simulink library "UserContent_lib"  (Simulink 7.8)
settings: Solver=ode45  SolverMode=SingleTasking  StartTime=0.0  StopTime=10.0  RelTol=1e-3
undefined symbols (not defined in the file): bias, ln, Timestep, u_gain_light, u_gain_moderate, u_gain_severe, v_gain_light, v_gain_moderate, v_gain_severe, w_gain_light, w_gain_moderate, w_gain_severe, WindDir, WindSpd
libraries: simulink x8
(part 1 of 2)
settings Model: Creator=Austin Murch  LastModifiedBy=decox

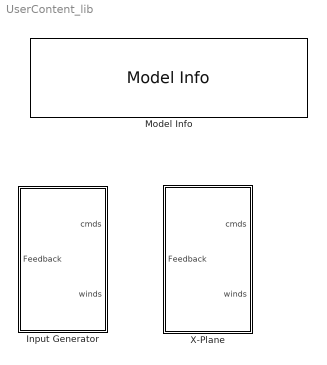
== system UserContent_lib ==
  Input Generator : Subsystem
  Model Info : simulink/Model-Wide Utilities/Model Info  InitialBlockCM=None  BlockCM=None  Frame=on  DisplayStringWithTags=|  HorizontalTextAlignment=Center  LeftAlignmentValue=0.5  SourceBlockDiagram=UserContent_lib  TagMaxNumber=20
      | - gtm_design Input Library -
      | 
      | Model Version: %<ModelVersion>
      | Last modifed by %<LastModifiedBy> on %<LastModificationDate>
  X-Plane : Subsystem

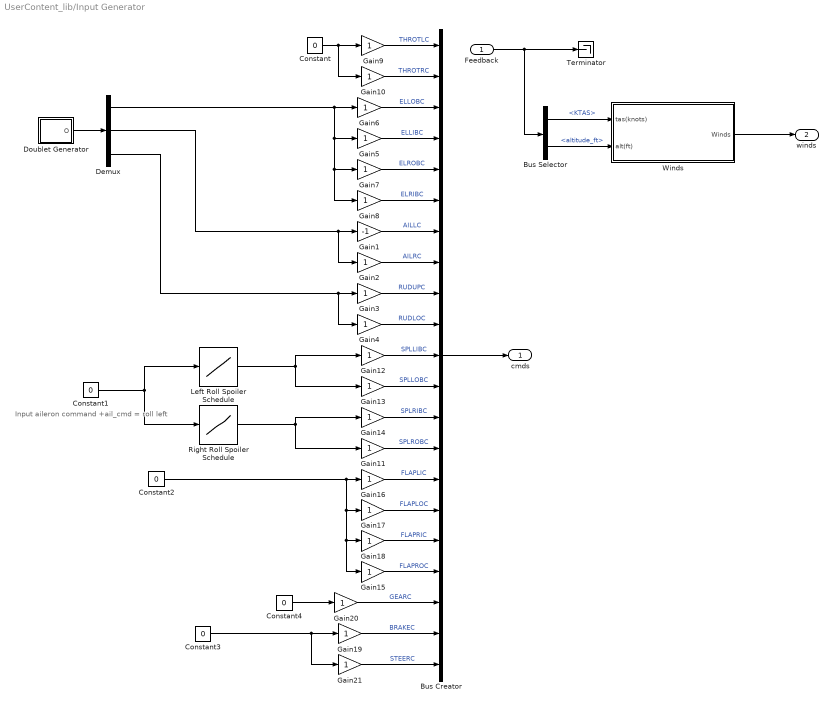
== system UserContent_lib/Input Generator ==
  note: Input aileron command
      | +ail_cmd = roll left
  Feedback : Inport
  Bus Creator : BusCreator  Inputs=21
  Bus Selector : BusSelector  OutputSignals=AirData.KTAS,AirData.altitude_ft
  Constant{,1..4} (5 alike) : Constant  Value=0
  Demux : Demux  Outputs=3
  Doublet Generator : Subsystem  mask(DoubletGenerator){timeon=[2 12 7], pulsewidth=[0.5 0.5 0.5], amplitude=[0 0 0]}
      mask prompts: timeon "Time Start"; pulsewidth "Pulse Duration"
      mask help:
      | Doublet Generator.
      | Ouputs doublet of specificed amplitude and duration.
      |
      | If start/duration/amplitude parameters are vectors, then output is multichannel.
      mask Display: plot([.1 .3 .3001 .4 .4001 .5  .5001 .7],[0 0 1 1 -1 -1 0 0])
  Gain1 : Gain  Gain=-1  SaturateOnIntegerOverflow=on  OutDataTypeStr=Inherit: Same as input  ParamDataTypeStr=Inherit: Same as input
  Gain{2..21} (20 alike) : Gain  SaturateOnIntegerOverflow=on  OutDataTypeStr=Inherit: Same as input  ParamDataTypeStr=Inherit: Same as input
  Left Roll Spoiler Schedule : Lookup  InputValues="[-20\t-11.76\t-2.36\t0\t2.36\t11.76\t20\t]"  Table=[0 0 0 0 0 9 45]  LookUpMeth=Interpolation-Use End Values
  Right Roll Spoiler Schedule : Lookup  InputValues="[-20\t-11.76\t-2.36\t0\t2.36\t11.76\t20\t]"  Table=[45 9 0 0 0 0 0]  LookUpMeth=Interpolation-Use End Values
  Terminator : Terminator
  Winds : Subsystem  mask(WindSource){WindSpeed_knots=WindSpd, WindDirection_deg=WindDir, level=None}
      mask prompts: WindSpeed_knots "Wind Speed (knots)"; WindDirection_deg "Wind Direction (deg)"; level "Turbulence Level"
      mask help:
      | Sets steady winds with wind speed and direction and
      | applies gust winds with selectable level of turbulence.
      mask StyleString: edit,edit,popup(None|Light|Moderate|Severe)
  cmds : Outport
  winds : Outport  Port=2
  wires:
  Winds/1(Winds) -> winds/1
  Constant1/1 -> Right Roll Spoiler Schedule/1, Left Roll Spoiler Schedule/1
  Right Roll Spoiler Schedule/1 -> Gain11/1, Gain14/1
  Left Roll Spoiler Schedule/1 -> Gain13/1, Gain12/1
  Gain12/1 -> Bus Creator/11  "SPLLIBC"
  Gain13/1 -> Bus Creator/12  "SPLLOBC"
  Gain14/1 -> Bus Creator/13  "SPLRIBC"
  Gain11/1 -> Bus Creator/14  "SPLROBC"
  Gain16/1 -> Bus Creator/15  "FLAPLIC"
  Gain17/1 -> Bus Creator/16  "FLAPLOC"
  Gain18/1 -> Bus Creator/17  "FLAPRIC"
  Gain15/1 -> Bus Creator/18  "FLAPROC"
  Gain9/1 -> Bus Creator/1  "THROTLC"
  Gain10/1 -> Bus Creator/2  "THROTRC"
  Gain5/1 -> Bus Creator/4  "ELLIBC"
  Gain6/1 -> Bus Creator/3  "ELLOBC"
  Gain7/1 -> Bus Creator/5  "ELROBC"
  Gain8/1 -> Bus Creator/6  "ELRIBC"
  Gain1/1 -> Bus Creator/7  "AILLC"
  Gain2/1 -> Bus Creator/8  "AILRC"
  Gain3/1 -> Bus Creator/9  "RUDUPC"
  Gain4/1 -> Bus Creator/10  "RUDLOC"
  Constant/1 -> Gain10/1, Gain9/1
  Constant2/1 -> Gain16/1, Gain17/1, Gain18/1, Gain15/1
  Doublet Generator/1(O) -> Demux/1
  Demux/2 -> Gain1/1, Gain2/1
  Demux/3 -> Gain3/1, Gain4/1
  Gain19/1 -> Bus Creator/20  "BRAKEC"
  Constant4/1 -> Gain20/1
  Constant3/1 -> Gain19/1, Gain21/1
  Demux/1 -> Gain6/1, Gain5/1, Gain7/1, Gain8/1
  Bus Creator/1 -> cmds/1
  Gain20/1 -> Bus Creator/19  "GEARC"
  Gain21/1 -> Bus Creator/21  "STEERC"
  Feedback/1 -> Terminator/1, Bus Selector/1
  Bus Selector/1 -> Winds/1(tas(knots))  "<KTAS>"
  Bus Selector/2 -> Winds/2(alt(ft))  "<altitude_ft>"

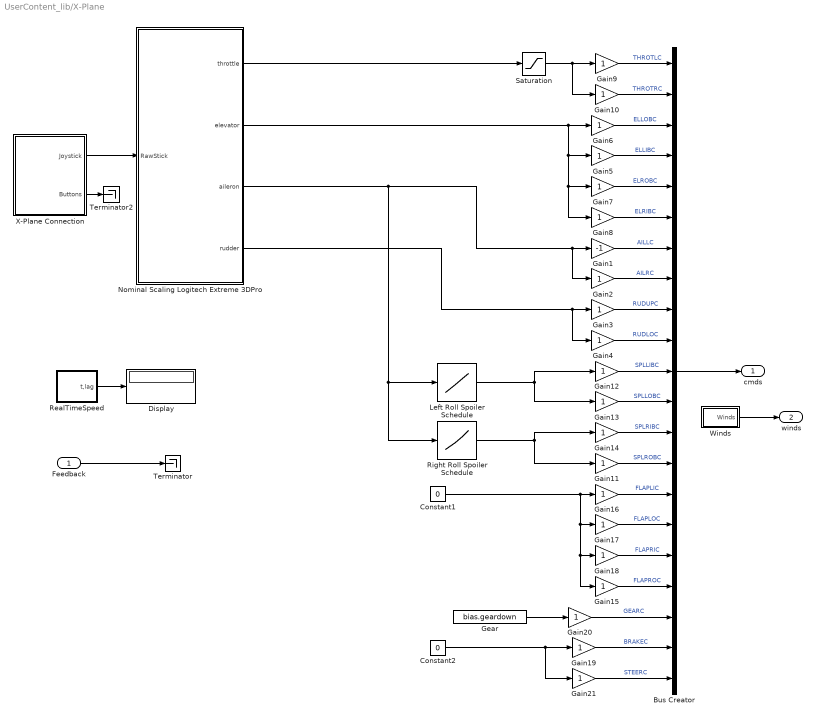
== system UserContent_lib/X-Plane ==
  Feedback : Inport
  Bus Creator : BusCreator  Inputs=21
  Constant1 : Constant  Value=0
  Constant2 : Constant  Value=0
  Display : Display
  Gain1 : Gain  Gain=-1  SaturateOnIntegerOverflow=on  OutDataTypeStr=Inherit: Same as input  ParamDataTypeStr=Inherit: Same as input
  Gain{2..21} (20 alike) : Gain  SaturateOnIntegerOverflow=on  OutDataTypeStr=Inherit: Same as input  ParamDataTypeStr=Inherit: Same as input
  Gear : Constant  Value=bias.geardown
  Left Roll Spoiler Schedule : Lookup  InputValues="[-20\t-11.76\t-2.36\t0\t2.36\t11.76\t20\t]"  Table=[0 0 0 0 0 9 45]  LookUpMeth=Interpolation-Use End Values
  Nominal Scaling Logitech Extreme 3DPro : Subsystem
  RealTimeSpeed : Subsystem
  Right Roll Spoiler Schedule : Lookup  InputValues="[-20\t-11.76\t-2.36\t0\t2.36\t11.76\t20\t]"  Table=[45 9 0 0 0 0 0]  LookUpMeth=Interpolation-Use End Values
  Saturation : Saturate  UpperLimit=100  LowerLimit=0
  Terminator : Terminator
  Terminator2 : Terminator
  Winds : Subsystem
  X-Plane Connection : Subsystem
  cmds : Outport
  winds : Outport  Port=2
  wires:
  Nominal Scaling Logitech Extreme 3DPro/1(throttle) -> Saturation/1
  Nominal Scaling Logitech Extreme 3DPro/2(elevator) -> Gain6/1, Gain5/1, Gain7/1, Gain8/1
  Nominal Scaling Logitech Extreme 3DPro/3(aileron) -> Right Roll Spoiler Schedule/1, Left Roll Spoiler Schedule/1, Gain1/1, Gain2/1
  Nominal Scaling Logitech Extreme 3DPro/4(rudder) -> Gain3/1, Gain4/1
  X-Plane Connection/2(Buttons) -> Terminator2/1
  Saturation/1 -> Gain10/1, Gain9/1
  RealTimeSpeed/1(t,lag) -> Display/1
  X-Plane Connection/1(Joystick) -> Nominal Scaling Logitech Extreme 3DPro/1(RawStick)
  Gain12/1 -> Bus Creator/11  "SPLLIBC"
  Gain13/1 -> Bus Creator/12  "SPLLOBC"
  Gain14/1 -> Bus Creator/13  "SPLRIBC"
  Gain11/1 -> Bus Creator/14  "SPLROBC"
  Gain16/1 -> Bus Creator/15  "FLAPLIC"
  Gain17/1 -> Bus Creator/16  "FLAPLOC"
  Gain18/1 -> Bus Creator/17  "FLAPRIC"
  Gain15/1 -> Bus Creator/18  "FLAPROC"
  Gain9/1 -> Bus Creator/1  "THROTLC"
  Gain10/1 -> Bus Creator/2  "THROTRC"
  Gain5/1 -> Bus Creator/4  "ELLIBC"
  Gain6/1 -> Bus Creator/3  "ELLOBC"
  Gain7/1 -> Bus Creator/5  "ELROBC"
  Gain8/1 -> Bus Creator/6  "ELRIBC"
  Gain1/1 -> Bus Creator/7  "AILLC"
  Gain2/1 -> Bus Creator/8  "AILRC"
  Gain3/1 -> Bus Creator/9  "RUDUPC"
  Gain4/1 -> Bus Creator/10  "RUDLOC"
  Constant1/1 -> Gain16/1, Gain17/1, Gain18/1, Gain15/1
  Gain19/1 -> Bus Creator/20  "BRAKEC"
  Gear/1 -> Gain20/1
  Constant2/1 -> Gain19/1, Gain21/1
  Bus Creator/1 -> cmds/1
  Gain20/1 -> Bus Creator/19  "GEARC"
  Gain21/1 -> Bus Creator/21  "STEERC"
  Left Roll Spoiler Schedule/1 -> Gain12/1, Gain13/1
  Right Roll Spoiler Schedule/1 -> Gain14/1, Gain11/1
  Feedback/1 -> Terminator/1
  Winds/1(Winds) -> winds/1

== system UserContent_lib/Input Generator/Doublet Generator ==
  Add : Sum  Inputs=+++
  DownStep : Step  Time=timeon+pulsewidth  After=-2  SampleTime=0
  Gain : Gain  Gain=amplitude
  UnStep : Step  Time=timeon+2*pulsewidth  SampleTime=0
  UpStep : Step  Time=timeon  SampleTime=0
  O : Outport
  wires:
  UpStep/1 -> Add/1
  DownStep/1 -> Add/2
  UnStep/1 -> Add/3
  Add/1 -> Gain/1
  Gain/1 -> O/1

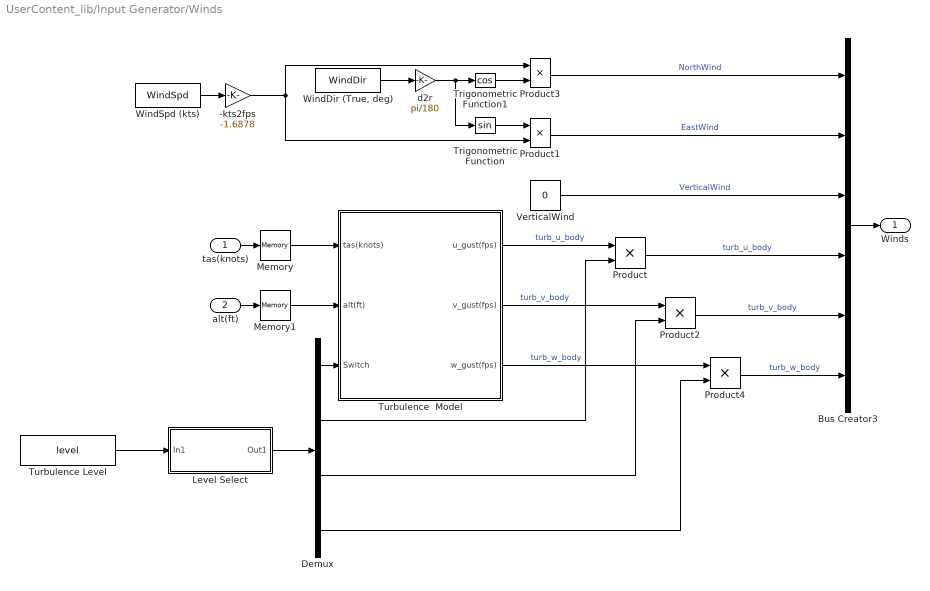
== system UserContent_lib/Input Generator/Winds ==
  tas(knots) : Inport
  alt(ft) : Inport  Port=2
  -kts2fps : Gain  Gain=-1.6878  SaturateOnIntegerOverflow=on  OutDataTypeStr=Inherit: Same as input  ParamDataTypeStr=Inherit: Same as input
  Bus Creator3 : BusCreator  Inputs=6
  Demux : Demux
  Level Select : Subsystem
  Memory : Memory  X0=70
  Memory1 : Memory  X0=1000
  Product : Product  RndMeth=Zero
  Product1 : Product  Inputs=**  SaturateOnIntegerOverflow=on  InputSameDT=on  OutDataTypeStr=Inherit: Same as first input
  Product2 : Product  RndMeth=Zero
  Product3 : Product  Inputs=**  SaturateOnIntegerOverflow=on  InputSameDT=on  OutDataTypeStr=Inherit: Same as first input
  Product4 : Product  RndMeth=Zero
  Trigonometric Function : Trigonometry
  Trigonometric Function1 : Trigonometry  Operator=cos
  Turbulence  Model : Subsystem
  Turbulence Level : Constant  Value=level
  VerticalWind : Constant  Value=0
  "WindDir (True, deg)" : Constant  Value=WindDir
  WindSpd (kts) : Constant  Value=WindSpd
  d2r : Gain  Gain=pi/180  SaturateOnIntegerOverflow=on  OutDataTypeStr=Inherit: Same as input  ParamDataTypeStr=Inherit: Same as input
  Winds : Outport
  wires:
  Demux/4 -> Product4/2
  Demux/3 -> Product2/2
  Demux/2 -> Product/2
  Demux/1 -> Turbulence  Model/3(Switch)
  Product3/1 -> Bus Creator3/1  "NorthWind"
  Product1/1 -> Bus Creator3/2  "EastWind"
  VerticalWind/1 -> Bus Creator3/3  "VerticalWind"
  Bus Creator3/1 -> Winds/1
  Trigonometric Function/1 -> Product1/1
  Trigonometric Function1/1 -> Product3/2
  d2r/1 -> Trigonometric Function1/1, Trigonometric Function/1
  "WindDir (True, deg)"/1 -> d2r/1
  WindSpd (kts)/1 -> -kts2fps/1
  -kts2fps/1 -> Product1/2, Product3/1
  Turbulence  Model/1(u_gust(fps)) -> Product/1  "turb_u_body"
  Turbulence  Model/2(v_gust(fps)) -> Product2/1  "turb_v_body"
  Turbulence  Model/3(w_gust(fps)) -> Product4/1  "turb_w_body"
  Product/1 -> Bus Creator3/4  "turb_u_body"
  Product2/1 -> Bus Creator3/5  "turb_v_body"
  Product4/1 -> Bus Creator3/6  "turb_w_body"
  tas(knots)/1 -> Memory/1
  alt(ft)/1 -> Memory1/1
  Memory/1 -> Turbulence  Model/1(tas(knots))
  Memory1/1 -> Turbulence  Model/2(alt(ft))
  Turbulence Level/1 -> Level Select/1(In1)
  Level Select/1(Out1) -> Demux/1

== system UserContent_lib/X-Plane/Nominal Scaling Logitech Extreme 3DPro ==
  RawStick : Inport
  Bias : Bias  Bias=[-1 -.5 -.5 -.5]
  Clock : Clock
  Constant : Constant  Value=zeros(4,1)
  Demux : Demux  Outputs=[4 -1]
  Demux1 : Demux
  Gain : Gain  Gain=[-100 -15 -15 -15]
  InitiallSupress Stick ToAllowTrim : Switch  Threshold=0.25
  Memory : Memory  X0=zeros(16,1)
  Selector : Selector  InputPortWidth=4  IndexOptions=Index vector (dialog)  Indices=[4 2 1 3]  OutputSizes=1
  Terminator3 : Terminator
  throttle : Outport
  elevator : Outport  Port=2
  aileron : Outport  Port=3
  rudder : Outport  Port=4
  wires:
  Demux1/4 -> rudder/1
  Demux1/3 -> aileron/1
  Demux1/2 -> elevator/1
  Demux1/1 -> throttle/1
  InitiallSupress Stick ToAllowTrim/1 -> Demux1/1
  Clock/1 -> InitiallSupress Stick ToAllowTrim/2
  Constant/1 -> InitiallSupress Stick ToAllowTrim/3
  Gain/1 -> InitiallSupress Stick ToAllowTrim/1
  Selector/1 -> Bias/1
  Bias/1 -> Gain/1
  RawStick/1 -> Memory/1
  Memory/1 -> Demux/1
  Demux/2 -> Terminator3/1
  Demux/1 -> Selector/1

== system UserContent_lib/X-Plane/RealTimeSpeed ==
  Clock : Clock
  Demux : Demux  Outputs=2
  Mux : Mux  Inputs=2
  S-Function : S-Function  FunctionName=RT_mex  EnableBusSupport=off
  Subtract : Sum  Inputs=+-
  t,lag : Outport
  wires:
  Mux/1 -> t,lag/1
  Subtract/1 -> Mux/2
  Demux/2 -> Subtract/2
  Demux/1 -> Mux/1, Subtract/1
  S-Function/1 -> Demux/1
  Clock/1 -> S-Function/1

== system UserContent_lib/X-Plane/Winds ==
  -kts2fps : Gain  Gain=-1.6878  SaturateOnIntegerOverflow=on  OutDataTypeStr=Inherit: Same as input  ParamDataTypeStr=Inherit: Same as input
  Bus Creator3 : BusCreator  Inputs=6
  Product1 : Product  Inputs=**  SaturateOnIntegerOverflow=on  InputSameDT=on  OutDataTypeStr=Inherit: Same as first input
  Product3 : Product  Inputs=**  SaturateOnIntegerOverflow=on  InputSameDT=on  OutDataTypeStr=Inherit: Same as first input
  Trigonometric Function : Trigonometry
  Trigonometric Function1 : Trigonometry  Operator=cos
  VerticalWind : Constant  Value=0
  "WindDir (True, deg)" : Constant  Value=WindDir
  WindSpd (kts) : Constant  Value=WindSpd
  d2r : Gain  Gain=pi/180  SaturateOnIntegerOverflow=on  OutDataTypeStr=Inherit: Same as input  ParamDataTypeStr=Inherit: Same as input
  turb_v_body : Constant  Value=0
  turb_v_body1 : Constant  Value=0
  turb_w_body : Constant  Value=0
  Winds : Outport
  wires:
  Product3/1 -> Bus Creator3/1  "NorthWind"
  Product1/1 -> Bus Creator3/2  "EastWind"
  VerticalWind/1 -> Bus Creator3/3  "VerticalWind"
  Bus Creator3/1 -> Winds/1
  Trigonometric Function/1 -> Product1/1
  Trigonometric Function1/1 -> Product3/2
  d2r/1 -> Trigonometric Function/1, Trigonometric Function1/1
  "WindDir (True, deg)"/1 -> d2r/1
  WindSpd (kts)/1 -> -kts2fps/1
  -kts2fps/1 -> Product3/1, Product1/2
  turb_v_body1/1 -> Bus Creator3/4  "turb_u_body"
  turb_v_body/1 -> Bus Creator3/5  "turb_v_body"
  turb_w_body/1 -> Bus Creator3/6  "turb_w_body"

== system UserContent_lib/X-Plane/X-Plane Connection ==
  Bus Selector1 : BusSelector  OutputSignals=AILR,ELRIB,RUDU,FLAPRIB,GEAR,BRAKE  OutputAsBus=on
  Bus Selector5 : BusSelector  OutputSignals=latitude,longitude,altitude,phi,theta,psi  OutputAsBus=on
  Bus Selector6 : BusSelector  OutputSignals=alpha,beta,tas  OutputAsBus=on
  Bus to Vector : BusToVector
  Bus to Vector1 : BusToVector
  Bus to Vector2 : BusToVector
  Xlink_fcn : Subsystem  mask(Xlink){HUDCell={'alpha','beta','Velocity'}}
      mask prompts: HUDCell "Lables for HUD, (cell array)"
      mask help:
      | Input Positions and Surfaces for X-Plane Visualization.
      |   Positions - [ Latitude, Longitude, Altitude, Roll, Pitch, Yaw] % degrees and ft.
      |   Surfaces  - [ Aileron, Elevator, Rudder, Flaps, Spoiler, GearDown] % deg and 0/1
      |
      | Output is Joysick axes and Button pushes.
      |   Joystick - First 16 axes
      |   Buttons  - 16 buttons as assigned to Xlink in X-Plane
      mask init:
      | if isempty(HUDCell) HUDCell=cell(6,1); end
      | HUDTextArray = uint8(zeros(90,1));
      | 
      | % loop through names, assign to string arrays
      | for i=1:min(length(HUDCell),6);
      |   if length(HUDCell{i})>14 HUDCell{i}=HUDCell{i}(1:14); end
      |   if length(HUDCell{i}>0),
      |     HUDTextArray((i-1)*15+1:(i-1)*15+length(HUDCell{i})) = uint8(HUDCell{i});
      |   end
      | end
  rad2deg : Gain  Gain=[180/pi 180/pi 1 180/pi 180/pi 180/pi]
  Joystick : Outport
  Buttons : Outport  Port=2
  wires:
  Bus Selector1/1 -> Bus to Vector1/1
  Bus to Vector1/1 -> Xlink_fcn/2(Surfaces)
  [SurfacePos] -> Bus Selector1/1
  rad2deg/1 -> Xlink_fcn/1(Positions)
  [EOM_State] -> Bus Selector5/1
  [AuxVars] -> Bus Selector6/1
  Bus Selector5/1 -> Bus to Vector2/1
  Xlink_fcn/2(Buttons) -> Buttons/1
  Xlink_fcn/1(Joystick) -> Joystick/1
  Bus Selector6/1 -> Bus to Vector/1
  Bus to Vector/1 -> Xlink_fcn/3(Overlay)
  Bus to Vector2/1 -> rad2deg/1

== system UserContent_lib/Input Generator/Winds/Level Select ==
  In1 : Inport
  Light : Constant  Value=[1 u_gain_light v_gain_light w_gain_light]
  Moderate : Constant  Value=[1 u_gain_moderate v_gain_moderate w_gain_moderate]
  Multiport Switch : MultiPortSwitch  Inputs=4  zeroidx=off
  Severe : Constant  Value=[1 u_gain_severe v_gain_severe w_gain_severe]
  Turbulence Off : Constant  Value=[0 0 0 0]
  Out1 : Outport
  wires:
  In1/1 -> Multiport Switch/1
  Turbulence Off/1 -> Multiport Switch/2
  Light/1 -> Multiport Switch/3
  Moderate/1 -> Multiport Switch/4
  Severe/1 -> Multiport Switch/5
  Multiport Switch/1 -> Out1/1

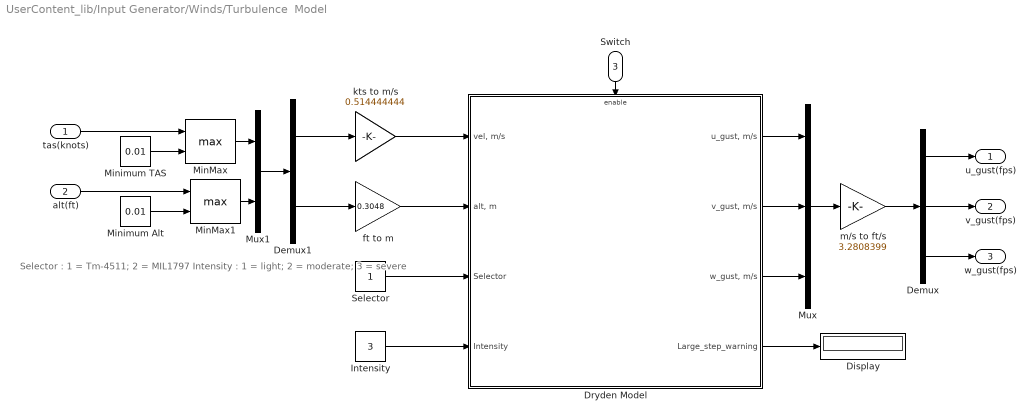
== system UserContent_lib/Input Generator/Winds/Turbulence  Model ==
  note: Selector :  1 = Tm-4511;  2 = MIL1797
      |             Intensity :  1 = light;  2 = moderate;  3 = severe
  tas(knots) : Inport
  alt(ft) : Inport  Port=2
  Switch : Inport  Port=3
  Demux : Demux  Outputs=3
  Demux1 : Demux  Outputs=2
  Display : Display
  Dryden Model : Subsystem  mask{longseed=3366+521, latseed=23+521, vertseed=1369+521, dt=Timestep, Step_warning_pct=.11}
      mask prompts: longseed "Longitudinal Random Number Seed"; latseed "Lateral Random Number Seed"; vertseed "Vertical Random Number Seed"; dt "Turbulence model time step, sec"; Step_warning_pct "Threshhold for stepsize warning (%)"
  Intensity : Constant  Value=3
  MinMax : MinMax  Function=max  Inputs=2
  MinMax1 : MinMax  Function=max  Inputs=2
  Minimum Alt : Constant  Value=0.01
  Minimum TAS : Constant  Value=0.01
  Mux : Mux  Inputs=3
  Mux1 : Mux  Inputs=2
  Selector : Constant
  ft to m : Gain  Gain=0.3048
  kts to m/s : Gain  Gain=0.514444444
  m/s to ft/s : Gain  Gain=3.2808399
  u_gust(fps) : Outport
  v_gust(fps) : Outport  Port=2
  w_gust(fps) : Outport  Port=3
  wires:
  Switch/1 -> Dryden Model/Enable
  Dryden Model/1("u_gust, m/s") -> Mux/1
  Dryden Model/2("v_gust, m/s") -> Mux/2
  Dryden Model/3("w_gust, m/s") -> Mux/3
  Demux/3 -> w_gust(fps)/1
  Demux/2 -> v_gust(fps)/1
  Demux/1 -> u_gust(fps)/1
  Dryden Model/4(Large_step_warning) -> Display/1
  Mux/1 -> m/s to ft/s/1
  m/s to ft/s/1 -> Demux/1
  MinMax1/1 -> Mux1/2
  MinMax/1 -> Mux1/1
  alt(ft)/1 -> MinMax1/1
  Minimum Alt/1 -> MinMax1/2
  Minimum TAS/1 -> MinMax/2
  tas(knots)/1 -> MinMax/1
  Mux1/1 -> Demux1/1
  Demux1/2 -> ft to m/1
  Demux1/1 -> kts to m/s/1
  Intensity/1 -> Dryden Model/4(Intensity)
  Selector/1 -> Dryden Model/3(Selector)
  ft to m/1 -> Dryden Model/2("alt, m")
  kts to m/s/1 -> Dryden Model/1("vel, m/s")

== system UserContent_lib/X-Plane/X-Plane Connection/Xlink_fcn ==
  note: Force Input to
      | dimension 6
  Positions : Inport
  Surfaces : Inport  Port=2
  Overlay : Inport  Port=3
  Demux : Demux  Outputs=[6 -1]
  Labels : Constant  Value=HUDTextArray  OutDataTypeStr=uint8
  Mux : Mux  Inputs=2
  S-Function : S-Function  FunctionName=SimulinkToXPlane  EnableBusSupport=off
  Saturation : Saturate  UpperLimit=[180*ones(5,1); 1]  LowerLimit=[-180*ones(5,1); 0]
  Signal Specification3 : SignalSpecification  Dimensions=6
  Terminator : Terminator
  zeros : Constant  Value=zeros(6,1)  OutDataTypeStr=double
  Joystick : Outport
  Buttons : Outport  Port=2
  wires:
  Demux/2 -> Terminator/1
  Demux/1 -> Signal Specification3/1
  Mux/1 -> Demux/1
  zeros/1 -> Mux/2
  Overlay/1 -> Mux/1
  Labels/1 -> S-Function/3
  Saturation/1 -> S-Function/2
  S-Function/2 -> Buttons/1
  Surfaces/1 -> Saturation/1
  S-Function/1 -> Joystick/1
  Positions/1 -> S-Function/1
  Signal Specification3/1 -> S-Function/4

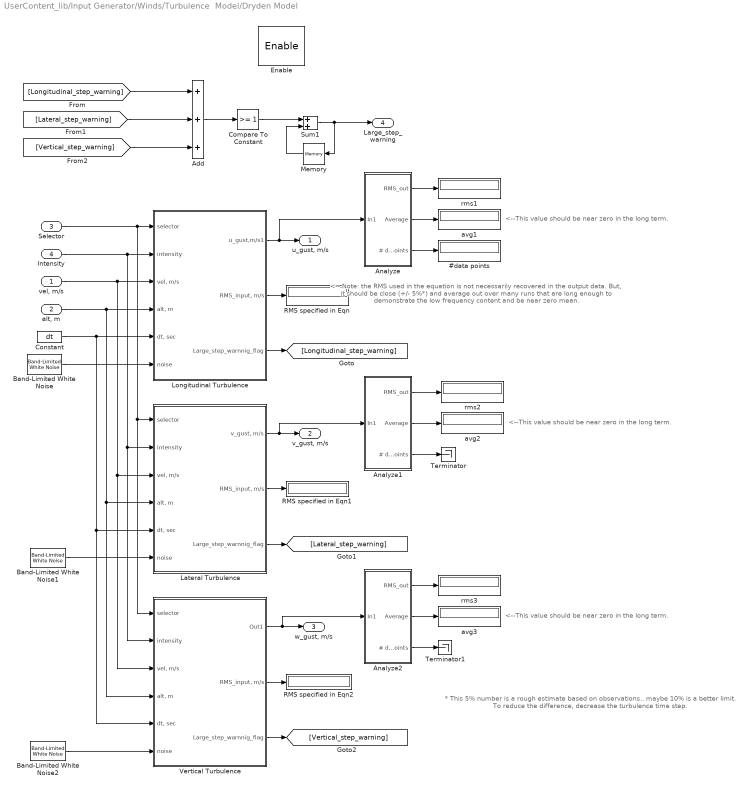
== system UserContent_lib/Input Generator/Winds/Turbulence  Model/Dryden Model ==
  note: * This 5% number is a rough estimate based on observations.. maybe 10% is a better limit.
      | To reduce the difference, decrease the turbulence time step.
  note: <--This value should be near zero in the long term.
  note: <--This value should be near zero in the long term.
  note: <--This value should be near zero in the long term.
  note: <-- Note: the RMS used in the equation is not necessarily recovered
      | in the output data.  But, it should be close (+/- 5%*) and  average out over
      | many runs that are long enough to demonstrate the low frequency
      | content and be near zero mean.
  "vel, m/s" : Inport
  "alt, m" : Inport  Port=2
  Selector : Inport  Port=3
  Intensity : Inport  Port=4
  Enable : EnablePort  StatesWhenEnabling=reset
  #data points : Display
  Add : Sum  Inputs=3
  Analyze : Subsystem
  Analyze1 : Subsystem
  Analyze2 : Subsystem
  Band-Limited White Noise : simulink/Sources/Band-Limited White Noise  Cov=dt  Ts=dt  seed=longseed
  Band-Limited White Noise1 : simulink/Sources/Band-Limited White Noise  Cov=dt  Ts=dt  seed=latseed
  Band-Limited White Noise2 : simulink/Sources/Band-Limited White Noise  Cov=dt  Ts=dt  seed=vertseed
  Compare To Constant : simulink/Logic and Bit Operations/Compare To Constant  relop=>=  const=1  OutDataTypeStr=uint8  ZeroCross=off
  Constant : Constant  Value=dt
  Lateral Turbulence : Subsystem
  Longitudinal Turbulence : Subsystem
  Memory : Memory
  RMS specified in Eqn : Display
  RMS specified in Eqn1 : Display
  RMS specified in Eqn2 : Display
  Sum1 : Sum  Inputs=2  SaturateOnIntegerOverflow=on
  Terminator : Terminator
  Terminator1 : Terminator
  Vertical Turbulence : Subsystem
  avg1 : Display
  avg2 : Display
  avg3 : Display
  rms1 : Display
  rms2 : Display
  rms3 : Display
  "u_gust, m/s" : Outport  OutputWhenDisabled=reset  InitialOutput=0
  "v_gust, m/s" : Outport  Port=2  OutputWhenDisabled=reset  InitialOutput=0
  "w_gust, m/s" : Outport  Port=3  OutputWhenDisabled=reset  InitialOutput=0
  Large_step_warning : Outport  Port=4  OutputWhenDisabled=reset  InitialOutput=0
  wires:
  Sum1/1 -> Memory/1, Large_step_warning/1
  Memory/1 -> Sum1/2
  Compare To Constant/1 -> Sum1/1
  Vertical Turbulence/3(Large_step_warnnig_flag) -> [Vertical_step_warning]
  Lateral Turbulence/3(Large_step_warnnig_flag) -> [Lateral_step_warning]
  Longitudinal Turbulence/3(Large_step_warnnig_flag) -> [Longitudinal_step_warning]
  [Lateral_step_warning] -> Add/2
  [Vertical_step_warning] -> Add/3
  [Longitudinal_step_warning] -> Add/1
  Add/1 -> Compare To Constant/1
  Band-Limited White Noise/1 -> Longitudinal Turbulence/6(noise)
  Analyze2/3(# data points) -> Terminator1/1
  Analyze1/3(# data points) -> Terminator/1
  Analyze/3(# data points) -> #data points/1
  Vertical Turbulence/2("RMS_input, m/s") -> RMS specified in Eqn2/1
  Lateral Turbulence/2("RMS_input, m/s") -> RMS specified in Eqn1/1
  Longitudinal Turbulence/2("RMS_input, m/s") -> RMS specified in Eqn/1
  Analyze2/2(Average) -> avg3/1
  Analyze2/1(RMS_out) -> rms3/1
  Vertical Turbulence/1(Out1) -> Analyze2/1(In1), "w_gust, m/s"/1
  Analyze1/2(Average) -> avg2/1
  Analyze1/1(RMS_out) -> rms2/1
  Lateral Turbulence/1("v_gust, m/s") -> Analyze1/1(In1), "v_gust, m/s"/1
  Analyze/2(Average) -> avg1/1
  Longitudinal Turbulence/1(u_gust,m/s1) -> Analyze/1(In1), "u_gust, m/s"/1
  Analyze/1(RMS_out) -> rms1/1
  Intensity/1 -> Lateral Turbulence/2(intensity), Vertical Turbulence/2(intensity), Longitudinal Turbulence/2(intensity)
  Band-Limited White Noise2/1 -> Vertical Turbulence/6(noise)
  Selector/1 -> Lateral Turbulence/1(selector), Vertical Turbulence/1(selector), Longitudinal Turbulence/1(selector)
  Band-Limited White Noise1/1 -> Lateral Turbulence/6(noise)
  Constant/1 -> Lateral Turbulence/5("dt, sec"), Vertical Turbulence/5("dt, sec"), Longitudinal Turbulence/5("dt, sec")
  "alt, m"/1 -> Lateral Turbulence/4("alt, m"), Vertical Turbulence/4("alt, m"), Longitudinal Turbulence/4("alt, m")
  "vel, m/s"/1 -> Lateral Turbulence/3("vel, m/s"), Vertical Turbulence/3("vel, m/s"), Longitudinal Turbulence/3("vel, m/s")

== system UserContent_lib/Input Generator/Winds/Turbulence  Model/Dryden Model/Analyze ==
  In1 : Inport
  Constant1 : Constant
  Constant3 : Constant  Value=0
  Constant5 : Constant  Value=dt
  Digital Clock1 : DigitalClock  SampleTime=dt
  Fcn : Fcn  Expr=sqrt(u)
  Memory : Memory
  Memory1 : Memory
  MinMax : MinMax  Function=max  Inputs=2
  Product : Product  SaturateOnIntegerOverflow=on  OutDataTypeStr=Inherit: Same as first input
  Product2 : Product  Inputs=/*  SaturateOnIntegerOverflow=on  OutDataTypeStr=Inherit: Same as first input
  Product3 : Product  Inputs=/*  SaturateOnIntegerOverflow=on  OutDataTypeStr=Inherit: Same as first input
  Product4 : Product  Inputs=/*  SaturateOnIntegerOverflow=on  OutDataTypeStr=Inherit: Same as first input
  Sum : Sum  Inputs=++-  SaturateOnIntegerOverflow=on
  Sum1 : Sum  Inputs=2  SaturateOnIntegerOverflow=on
  RMS_out : Outport
  Average : Outport  Port=2
  # data points : Outport  Port=3
  wires:
  MinMax/1 -> Product2/1, Product4/1
  Constant1/1 -> MinMax/2
  In1/1 -> Sum1/1, Product/1, Product/2
  Product/1 -> Sum/2
  Sum/1 -> Memory1/1, Product2/2
  Sum1/1 -> Memory/1, Product4/2
  Product2/1 -> Fcn/1
  Memory/1 -> Sum1/2
  Memory1/1 -> Sum/1
  Constant3/1 -> Sum/3
  Constant5/1 -> Product3/1
  Digital Clock1/1 -> Product3/2
  Product3/1 -> MinMax/1, # data points/1
  Fcn/1 -> RMS_out/1
  Product4/1 -> Average/1

== system UserContent_lib/Input Generator/Winds/Turbulence  Model/Dryden Model/Analyze1 ==
  In1 : Inport
  Constant1 : Constant
  Constant3 : Constant  Value=0
  Constant5 : Constant  Value=dt
  Digital Clock1 : DigitalClock  SampleTime=dt
  Fcn : Fcn  Expr=sqrt(u)
  Memory : Memory
  Memory1 : Memory
  MinMax : MinMax  Function=max  Inputs=2
  Product : Product  SaturateOnIntegerOverflow=on  OutDataTypeStr=Inherit: Same as first input
  Product2 : Product  Inputs=/*  SaturateOnIntegerOverflow=on  OutDataTypeStr=Inherit: Same as first input
  Product3 : Product  Inputs=/*  SaturateOnIntegerOverflow=on  OutDataTypeStr=Inherit: Same as first input
  Product4 : Product  Inputs=/*  SaturateOnIntegerOverflow=on  OutDataTypeStr=Inherit: Same as first input
  Sum : Sum  Inputs=++-  SaturateOnIntegerOverflow=on
  Sum1 : Sum  Inputs=2  SaturateOnIntegerOverflow=on
  RMS_out : Outport
  Average : Outport  Port=2
  # data points : Outport  Port=3
  wires:
  Product4/1 -> Average/1
  Fcn/1 -> RMS_out/1
  Product3/1 -> # data points/1, MinMax/1
  Digital Clock1/1 -> Product3/2
  Constant5/1 -> Product3/1
  Constant3/1 -> Sum/3
  Memory1/1 -> Sum/1
  Memory/1 -> Sum1/2
  Product2/1 -> Fcn/1
  Sum1/1 -> Product4/2, Memory/1
  Sum/1 -> Product2/2, Memory1/1
  Product/1 -> Sum/2
  In1/1 -> Product/2, Product/1, Sum1/1
  Constant1/1 -> MinMax/2
  MinMax/1 -> Product4/1, Product2/1

== system UserContent_lib/Input Generator/Winds/Turbulence  Model/Dryden Model/Analyze2 ==
  In1 : Inport
  Constant1 : Constant
  Constant3 : Constant  Value=0
  Constant5 : Constant  Value=dt
  Digital Clock1 : DigitalClock  SampleTime=dt
  Fcn : Fcn  Expr=sqrt(u)
  Memory : Memory
  Memory1 : Memory
  MinMax : MinMax  Function=max  Inputs=2
  Product : Product  SaturateOnIntegerOverflow=on  OutDataTypeStr=Inherit: Same as first input
  Product2 : Product  Inputs=/*  SaturateOnIntegerOverflow=on  OutDataTypeStr=Inherit: Same as first input
  Product3 : Product  Inputs=/*  SaturateOnIntegerOverflow=on  OutDataTypeStr=Inherit: Same as first input
  Product4 : Product  Inputs=/*  SaturateOnIntegerOverflow=on  OutDataTypeStr=Inherit: Same as first input
  Sum : Sum  Inputs=++-  SaturateOnIntegerOverflow=on
  Sum1 : Sum  Inputs=2  SaturateOnIntegerOverflow=on
  RMS_out : Outport
  Average : Outport  Port=2
  # data points : Outport  Port=3
  wires:
  MinMax/1 -> Product2/1, Product4/1
  Constant1/1 -> MinMax/2
  In1/1 -> Sum1/1, Product/1, Product/2
  Product/1 -> Sum/2
  Sum/1 -> Memory1/1, Product2/2
  Sum1/1 -> Memory/1, Product4/2
  Product2/1 -> Fcn/1
  Memory/1 -> Sum1/2
  Memory1/1 -> Sum/1
  Constant3/1 -> Sum/3
  Constant5/1 -> Product3/1
  Digital Clock1/1 -> Product3/2
  Product3/1 -> MinMax/1, # data points/1
  Fcn/1 -> RMS_out/1
  Product4/1 -> Average/1

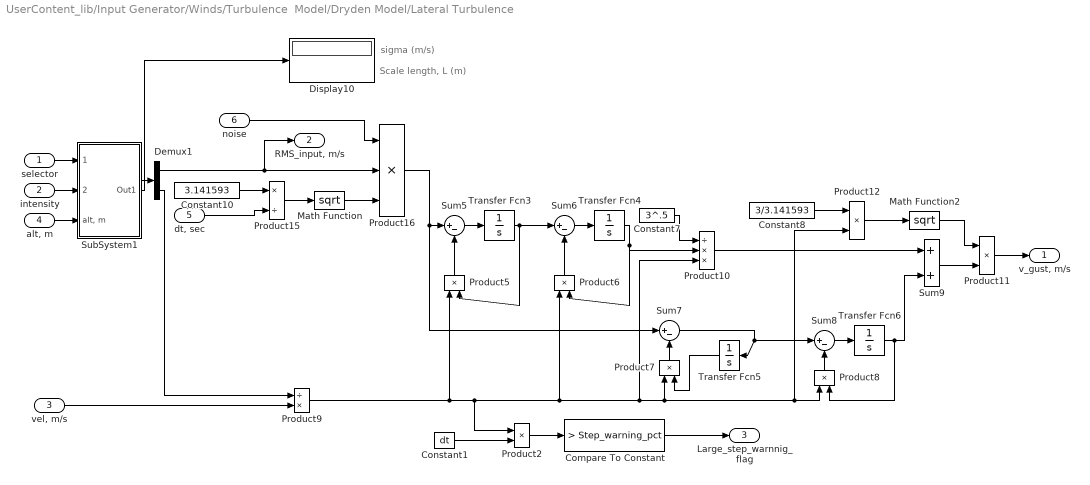
== system UserContent_lib/Input Generator/Winds/Turbulence  Model/Dryden Model/Lateral Turbulence ==
  note: Scale length, L (m)
  note: sigma (m/s)
  selector : Inport
  intensity : Inport  Port=2
  "vel, m/s" : Inport  Port=3
  "alt, m" : Inport  Port=4
  "dt, sec" : Inport  Port=5
  noise : Inport  Port=6
  Compare To Constant : simulink/Logic and Bit Operations/Compare To Constant  relop=>  const=Step_warning_pct  OutDataTypeStr=uint8  ZeroCross=off
  Constant1 : Constant  Value=dt
  Constant10 : Constant  Value=3.141593
  Constant7 : Constant  Value=3^.5
  Constant8 : Constant  Value=3/3.141593
  Demux1 : Demux  Outputs=2
  Display10 : Display
  Math Function : Math  Operator=sqrt  SaturateOnIntegerOverflow=on
  Math Function2 : Math  Operator=sqrt  SaturateOnIntegerOverflow=on
  Product10 : Product  Inputs=/**  SaturateOnIntegerOverflow=on  InputSameDT=on  OutDataTypeStr=Inherit: Same as first input
  Product11 : Product  Inputs=**  SaturateOnIntegerOverflow=on  InputSameDT=on  OutDataTypeStr=Inherit: Same as first input
  Product12 : Product  Inputs=**  SaturateOnIntegerOverflow=on  InputSameDT=on  OutDataTypeStr=Inherit: Same as first input
  Product15 : Product  Inputs=*/  SaturateOnIntegerOverflow=on  InputSameDT=on  OutDataTypeStr=Inherit: Same as first input
  Product16 : Product  Inputs=***  SaturateOnIntegerOverflow=on  InputSameDT=on  OutDataTypeStr=Inherit: Same as first input
  Product{2,5..8} (5 alike) : Product  SaturateOnIntegerOverflow=on  InputSameDT=on  OutDataTypeStr=Inherit: Same as first input
  Product9 : Product  Inputs=/*  SaturateOnIntegerOverflow=on  InputSameDT=on  OutDataTypeStr=Inherit: Same as first input
  SubSystem1 : Subsystem
  Sum{5..8} (4 alike) : Sum  Inputs=|+-  SaturateOnIntegerOverflow=on  InputSameDT=on  OutDataTypeStr=Inherit: Same as first input
  Sum9 : Sum  Inputs=2  SaturateOnIntegerOverflow=on  InputSameDT=on  OutDataTypeStr=Inherit: Same as first input
  Transfer Fcn{3..6} (4 alike) : TransferFcn  Numerator=1  Denominator=[1 0]
  "v_gust, m/s" : Outport
  "RMS_input, m/s" : Outport  Port=2
  Large_step_warnnig_flag : Outport  Port=3
  wires:
  Compare To Constant/1 -> Large_step_warnnig_flag/1
  Product2/1 -> Compare To Constant/1
  Constant1/1 -> Product2/2
  Math Function/1 -> Product16/3
  intensity/1 -> SubSystem1/2(intensity)
  selector/1 -> SubSystem1/1(selector)
  "alt, m"/1 -> SubSystem1/3("alt, m")
  Demux1/2 -> Product9/1
  SubSystem1/1(Out1) -> Display10/1, Demux1/1
  Product16/1 -> Sum7/1, Sum5/1
  Demux1/1 -> Product16/2, "RMS_input, m/s"/1
  "dt, sec"/1 -> Product15/2
  Product9/1 -> Product2/1, Product10/3, Product12/2, Product8/1, Product7/1, Product6/1, Product5/1
  "vel, m/s"/1 -> Product9/2
  Product12/1 -> Math Function2/1
  Constant8/1 -> Product12/1
  Math Function2/1 -> Product11/1
  Sum9/1 -> Product11/2
  Constant7/1 -> Product10/1
  Product10/1 -> Sum9/1
  Transfer Fcn6/1 -> Sum9/2, Product8/2
  Sum7/1 -> Sum8/1, Transfer Fcn5/1
  Product8/1 -> Sum8/2
  Sum8/1 -> Transfer Fcn6/1
  Product7/1 -> Sum7/2
  Transfer Fcn5/1 -> Product7/2
  Transfer Fcn4/1 -> Product10/2, Product6/2
  Transfer Fcn3/1 -> Sum6/1, Product5/2
  Product6/1 -> Sum6/2
  Sum6/1 -> Transfer Fcn4/1
  Sum5/1 -> Transfer Fcn3/1
  Product5/1 -> Sum5/2
  noise/1 -> Product16/1
  Constant10/1 -> Product15/1
  Product15/1 -> Math Function/1
  Product11/1 -> "v_gust, m/s"/1

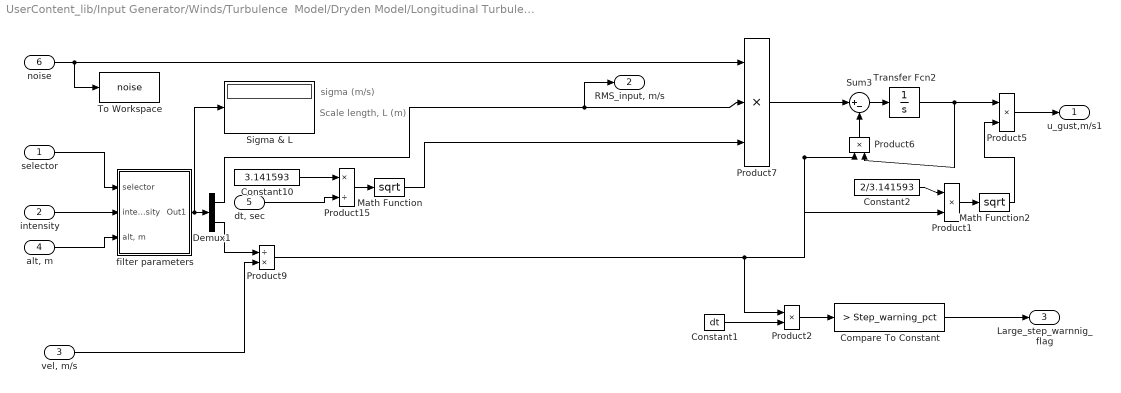
== system UserContent_lib/Input Generator/Winds/Turbulence  Model/Dryden Model/Longitudinal Turbulence ==
  note: Scale length, L (m)
  note: sigma (m/s)
  selector : Inport
  intensity : Inport  Port=2
  "vel, m/s" : Inport  Port=3
  "alt, m" : Inport  Port=4
  "dt, sec" : Inport  Port=5
  noise : Inport  Port=6
  Compare To Constant : simulink/Logic and Bit Operations/Compare To Constant  relop=>  const=Step_warning_pct  OutDataTypeStr=uint8  ZeroCross=off
  Constant1 : Constant  Value=dt
  Constant10 : Constant  Value=3.141593
  Constant2 : Constant  Value=2/3.141593
  Demux1 : Demux  Outputs=2
  Math Function : Math  Operator=sqrt  SaturateOnIntegerOverflow=on
  Math Function2 : Math  Operator=sqrt  SaturateOnIntegerOverflow=on
  Product1 : Product  Inputs=**  SaturateOnIntegerOverflow=on  InputSameDT=on  OutDataTypeStr=Inherit: Same as first input
  Product15 : Product  Inputs=*/  SaturateOnIntegerOverflow=on  InputSameDT=on  OutDataTypeStr=Inherit: Same as first input
  Product2 : Product  SaturateOnIntegerOverflow=on  InputSameDT=on  OutDataTypeStr=Inherit: Same as first input
  Product5 : Product  Inputs=**  SaturateOnIntegerOverflow=on  InputSameDT=on  OutDataTypeStr=Inherit: Same as first input
  Product6 : Product  SaturateOnIntegerOverflow=on  InputSameDT=on  OutDataTypeStr=Inherit: Same as first input
  Product7 : Product  Inputs=***  SaturateOnIntegerOverflow=on  InputSameDT=on  OutDataTypeStr=Inherit: Same as first input
  Product9 : Product  Inputs=/*  SaturateOnIntegerOverflow=on  InputSameDT=on  OutDataTypeStr=Inherit: Same as first input
  Sigma & L : Display
  Sum3 : Sum  Inputs=|+-  SaturateOnIntegerOverflow=on  InputSameDT=on  OutDataTypeStr=Inherit: Same as first input
  To Workspace : ToWorkspace  VariableName=noise  SampleTime=-1  SaveFormat=Array
  Transfer Fcn2 : TransferFcn  Numerator=1  Denominator=[1 0]
  filter parameters : Subsystem
  u_gust,m/s1 : Outport
  "RMS_input, m/s" : Outport  Port=2
  Large_step_warnnig_flag : Outport  Port=3
  wires:
  Compare To Constant/1 -> Large_step_warnnig_flag/1
  Product2/1 -> Compare To Constant/1
  Constant1/1 -> Product2/2
  Product7/1 -> Sum3/1
  Product6/1 -> Sum3/2
  Product5/1 -> u_gust,m/s1/1
  Math Function2/1 -> Product5/2
  Product1/1 -> Math Function2/1
  Constant2/1 -> Product1/1
  Sum3/1 -> Transfer Fcn2/1
  Transfer Fcn2/1 -> Product5/1, Product6/2
  intensity/1 -> filter parameters/2(intensity)
  Demux1/1 -> "RMS_input, m/s"/1, Product7/2
  Demux1/2 -> Product9/1
  filter parameters/1(Out1) -> Demux1/1, Sigma & L/1
  noise/1 -> Product7/1, To Workspace/1
  "dt, sec"/1 -> Product15/2
  "vel, m/s"/1 -> Product9/2
  Constant10/1 -> Product15/1
  Product9/1 -> Product2/1, Product1/2, Product6/1
  Math Function/1 -> Product7/3
  Product15/1 -> Math Function/1
  selector/1 -> filter parameters/1(selector)
  "alt, m"/1 -> filter parameters/3("alt, m")

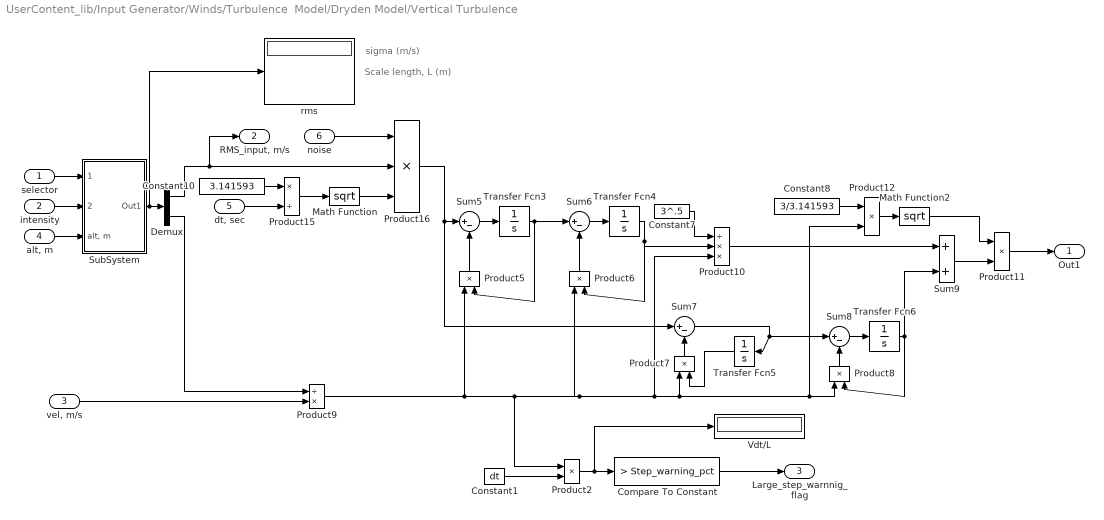
== system UserContent_lib/Input Generator/Winds/Turbulence  Model/Dryden Model/Vertical Turbulence ==
  note: Scale length, L (m)
  note: sigma (m/s)
  selector : Inport
  intensity : Inport  Port=2
  "vel, m/s" : Inport  Port=3
  "alt, m" : Inport  Port=4
  "dt, sec" : Inport  Port=5
  noise : Inport  Port=6
  Compare To Constant : simulink/Logic and Bit Operations/Compare To Constant  relop=>  const=Step_warning_pct  OutDataTypeStr=uint8  ZeroCross=off
  Constant1 : Constant  Value=dt
  Constant10 : Constant  Value=3.141593
  Constant7 : Constant  Value=3^.5
  Constant8 : Constant  Value=3/3.141593
  Demux : Demux  Outputs=2
  Math Function : Math  Operator=sqrt  SaturateOnIntegerOverflow=on
  Math Function2 : Math  Operator=sqrt  SaturateOnIntegerOverflow=on
  Product10 : Product  Inputs=/**  SaturateOnIntegerOverflow=on  InputSameDT=on  OutDataTypeStr=Inherit: Same as first input
  Product11 : Product  Inputs=**  SaturateOnIntegerOverflow=on  InputSameDT=on  OutDataTypeStr=Inherit: Same as first input
  Product12 : Product  Inputs=**  SaturateOnIntegerOverflow=on  InputSameDT=on  OutDataTypeStr=Inherit: Same as first input
  Product15 : Product  Inputs=*/  SaturateOnIntegerOverflow=on  InputSameDT=on  OutDataTypeStr=Inherit: Same as first input
  Product16 : Product  Inputs=***  SaturateOnIntegerOverflow=on  InputSameDT=on  OutDataTypeStr=Inherit: Same as first input
  Product{2,5..8} (5 alike) : Product  SaturateOnIntegerOverflow=on  InputSameDT=on  OutDataTypeStr=Inherit: Same as first input
  Product9 : Product  Inputs=/*  SaturateOnIntegerOverflow=on  InputSameDT=on  OutDataTypeStr=Inherit: Same as first input
  SubSystem : Subsystem
  Sum{5..8} (4 alike) : Sum  Inputs=|+-  SaturateOnIntegerOverflow=on  InputSameDT=on  OutDataTypeStr=Inherit: Same as first input
  Sum9 : Sum  Inputs=2  SaturateOnIntegerOverflow=on  InputSameDT=on  OutDataTypeStr=Inherit: Same as first input
  Transfer Fcn{3..6} (4 alike) : TransferFcn  Numerator=1  Denominator=[1 0]
  Vdt/L : Display
  rms : Display
  Out1 : Outport
  "RMS_input, m/s" : Outport  Port=2
  Large_step_warnnig_flag : Outport  Port=3
  wires:
  Compare To Constant/1 -> Large_step_warnnig_flag/1
  Product2/1 -> Vdt/L/1, Compare To Constant/1
  Constant1/1 -> Product2/2
  intensity/1 -> SubSystem/2("intensity ")
  selector/1 -> SubSystem/1(selector)
  "alt, m"/1 -> SubSystem/3("alt, m")
  SubSystem/1(Out1) -> rms/1, Demux/1
  Demux/2 -> Product9/1
  Demux/1 -> "RMS_input, m/s"/1, Product16/2
  noise/1 -> Product16/1
  Product16/1 -> Sum7/1, Sum5/1
  "dt, sec"/1 -> Product15/2
  Math Function/1 -> Product16/3
  Product9/1 -> Product2/1, Product10/3, Product12/2, Product8/1, Product7/1, Product6/1, Product5/1
  "vel, m/s"/1 -> Product9/2
  Product12/1 -> Math Function2/1
  Constant8/1 -> Product12/1
  Math Function2/1 -> Product11/1
  Sum9/1 -> Product11/2
  Constant7/1 -> Product10/1
  Product10/1 -> Sum9/1
  Transfer Fcn6/1 -> Sum9/2, Product8/2
  Sum7/1 -> Sum8/1, Transfer Fcn5/1
  Product8/1 -> Sum8/2
  Sum8/1 -> Transfer Fcn6/1
  Product7/1 -> Sum7/2
  Transfer Fcn5/1 -> Product7/2
  Transfer Fcn4/1 -> Product10/2, Product6/2
  Transfer Fcn3/1 -> Sum6/1, Product5/2
  Product6/1 -> Sum6/2
  Sum6/1 -> Transfer Fcn4/1
  Sum5/1 -> Transfer Fcn3/1
  Product5/1 -> Sum5/2
  Constant10/1 -> Product15/1
  Product15/1 -> Math Function/1
  Product11/1 -> Out1/1

== system UserContent_lib/Input Generator/Winds/Turbulence  Model/Dryden Model/Lateral Turbulence/SubSystem1 ==
  note: light=1
      | moderate=2
      | severe=3
  selector : Inport
  intensity : Inport  Port=2
  "alt, m" : Inport  Port=3
  L^.333 : Fcn  Expr=u(1)^(1/3)
  L^.334 : Fcn  Expr=u(1)^(1/3)
  Lv : Scope
  "MIL-STD-1797A APPENDIX A " : Subsystem
  Multiport Switch : MultiPortSwitch  Inputs=2  zeroidx=off  SaturateOnIntegerOverflow=on  InputSameDT=on
  Mux{,1..4} (5 alike) : Mux  Inputs=2
  Product1 : Product  Inputs=*/  SaturateOnIntegerOverflow=on  InputSameDT=on  OutDataTypeStr=Inherit: Same as first input
  Product2 : Product  Inputs=*/  SaturateOnIntegerOverflow=on  InputSameDT=on  OutDataTypeStr=Inherit: Same as first input
  Tm-4511 severe data : Subsystem
  sigma / Lw^.333 : Scope
  sigmav : Scope
  Out1 : Outport
  wires:
  L^.333/1 -> Product1/2
  Product1/1 -> Mux4/1
  Product2/1 -> Mux4/2
  Mux4/1 -> sigma / Lw^.333/1
  L^.334/1 -> Product2/2
  "MIL-STD-1797A APPENDIX A "/2("scale length, m") -> L^.334/1, Mux3/2, Mux1/2
  Tm-4511 severe data/2("scale length, m") -> L^.333/1, Mux3/1, Mux/2
  "MIL-STD-1797A APPENDIX A "/1("sigma, m/s") -> Product2/1, Mux2/2, Mux1/1
  Mux2/1 -> sigmav/1
  Mux3/1 -> Lv/1
  Mux1/1 -> Multiport Switch/3
  intensity/1 -> Tm-4511 severe data/2(intensity), "MIL-STD-1797A APPENDIX A "/2(intensity)
  "alt, m"/1 -> "MIL-STD-1797A APPENDIX A "/1("alt, m"), Tm-4511 severe data/1("alt, m")
  Mux/1 -> Multiport Switch/2
  Tm-4511 severe data/1("sigma, m/s") -> Product1/1, Mux2/1, Mux/1
  Multiport Switch/1 -> Out1/1
  selector/1 -> Multiport Switch/1

== system UserContent_lib/Input Generator/Winds/Turbulence  Model/Dryden Model/Longitudinal Turbulence/filter parameters ==
  note: light=1
      | moderate=2
      | severe=3
  selector : Inport
  intensity : Inport  Port=2
  "alt, m" : Inport  Port=3
  L^.333 : Fcn  Expr=u(1)^(1/3)
  L^.334 : Fcn  Expr=u(1)^(1/3)
  Lu : Scope
  "MIL-STD-1797A APPENDIX A " : Subsystem
  Multiport Switch : MultiPortSwitch  Inputs=2  zeroidx=off  SaturateOnIntegerOverflow=on  InputSameDT=on
  Mux{,1..4} (5 alike) : Mux  Inputs=2
  Product1 : Product  Inputs=*/  SaturateOnIntegerOverflow=on  InputSameDT=on  OutDataTypeStr=Inherit: Same as first input
  Product2 : Product  Inputs=*/  SaturateOnIntegerOverflow=on  InputSameDT=on  OutDataTypeStr=Inherit: Same as first input
  Tm-4511 severe data : Subsystem
  sigma / Lu^.333 : Scope
      settings: YMin=0  YMax=60
  sigma u : Scope
      settings: YMin=2  YMax=5.75
  Out1 : Outport
  wires:
  L^.334/1 -> Product2/2
  L^.333/1 -> Product1/2
  Product1/1 -> Mux4/1
  Product2/1 -> Mux4/2
  Mux4/1 -> sigma / Lu^.333/1
  "MIL-STD-1797A APPENDIX A "/2("scale length, m") -> L^.334/1, Mux3/2, Mux1/2
  Tm-4511 severe data/2("scale length, m") -> L^.333/1, Mux3/1, Mux/2
  "MIL-STD-1797A APPENDIX A "/1("sigma, m/s") -> Product2/1, Mux2/2, Mux1/1
  Mux2/1 -> sigma u/1
  Mux3/1 -> Lu/1
  intensity/1 -> Tm-4511 severe data/2(intensity), "MIL-STD-1797A APPENDIX A "/2(intensity)
  "alt, m"/1 -> "MIL-STD-1797A APPENDIX A "/1("alt, m"), Tm-4511 severe data/1("alt, m")
  Mux1/1 -> Multiport Switch/3
  Mux/1 -> Multiport Switch/2
  Tm-4511 severe data/1("sigma, m/s") -> Mux/1, Product1/1, Mux2/1
  Multiport Switch/1 -> Out1/1
  selector/1 -> Multiport Switch/1

== system UserContent_lib/Input Generator/Winds/Turbulence  Model/Dryden Model/Vertical Turbulence/SubSystem ==
  note: light=1
      | moderate=2
      | severe=3
  selector : Inport
  "intensity " : Inport  Port=2
  "alt, m" : Inport  Port=3
  L^.333 : Fcn  Expr=u(1)^(1/3)
  L^.334 : Fcn  Expr=u(1)^(1/3)
  Lw : Scope
  "MIL-STD-1797A APPENDIX A " : Subsystem
  Multiport Switch : MultiPortSwitch  Inputs=2  zeroidx=off  SaturateOnIntegerOverflow=on  InputSameDT=on
  Mux{,1..4} (5 alike) : Mux  Inputs=2
  Product1 : Product  Inputs=*/  SaturateOnIntegerOverflow=on  InputSameDT=on  OutDataTypeStr=Inherit: Same as first input
  Product2 : Product  Inputs=*/  SaturateOnIntegerOverflow=on  InputSameDT=on  OutDataTypeStr=Inherit: Same as first input
  Tm-4511 severe data : Subsystem
  sigma / Lw^.333 : Scope
  sigma w : Scope
      settings: YMin=0.75  YMax=5.75
  Out1 : Outport
  wires:
  L^.334/1 -> Product2/2
  L^.333/1 -> Product1/2
  Product1/1 -> Mux4/1
  Product2/1 -> Mux4/2
  Mux4/1 -> sigma / Lw^.333/1
  Mux2/1 -> sigma w/1
  Mux3/1 -> Lw/1
  "MIL-STD-1797A APPENDIX A "/2("scale length, m") -> L^.334/1, Mux3/2, Mux1/2
  Tm-4511 severe data/2("scale length, m") -> L^.333/1, Mux3/1, Mux/2
  "MIL-STD-1797A APPENDIX A "/1("sigma, m/s") -> Product2/1, Mux2/2, Mux1/1
  Mux1/1 -> Multiport Switch/3
  Mux/1 -> Multiport Switch/2
  "intensity "/1 -> Tm-4511 severe data/2(intensity), "MIL-STD-1797A APPENDIX A "/2(intensity)
  "alt, m"/1 -> "MIL-STD-1797A APPENDIX A "/1("alt, m"), Tm-4511 severe data/1("alt, m")
  Tm-4511 severe data/1("sigma, m/s") -> Product1/1, Mux2/1, Mux/1
  Multiport Switch/1 -> Out1/1
  selector/1 -> Multiport Switch/1

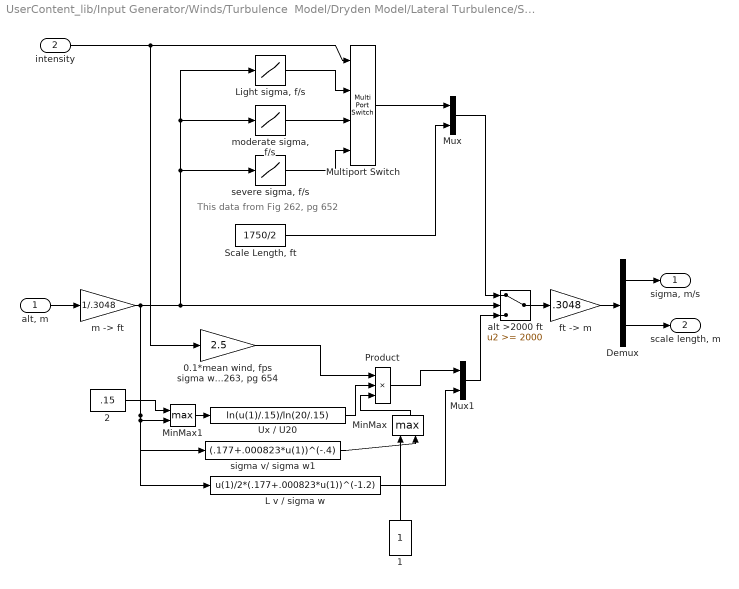
== system UserContent_lib/Input Generator/Winds/Turbulence  Model/Dryden Model/Lateral Turbulence/SubSystem1/MIL-STD-1797A APPENDIX A  ==
  note: This data from Fig 262, pg 652
  "alt, m" : Inport
  intensity : Inport  Port=2
  "0.1*mean wind, fps sigma w = to 2.5f/s * intensity Fig 263, pg 654" : Gain  Gain=2.5  SaturateOnIntegerOverflow=on  OutDataTypeStr=Inherit: Same as input  ParamDataTypeStr=Inherit: Same as input
  1 : Constant
  2 : Constant  Value=.15
  Demux : Demux  Outputs=2
  L v / sigma w : Fcn  Expr=u(1)/2*(.177+.000823*u(1))^(-1.2)
  "Light sigma, f/s" : Lookup  InputValues=[2000 9000 18000 100000]  Table=[5 5 3 3]  SaturateOnIntegerOverflow=on
  MinMax : MinMax  Function=max  Inputs=2  SaturateOnIntegerOverflow=on  InputSameDT=on
  MinMax1 : MinMax  Function=max  Inputs=2  SaturateOnIntegerOverflow=on  InputSameDT=on
  Multiport Switch : MultiPortSwitch  zeroidx=off  SaturateOnIntegerOverflow=on  InputSameDT=on
  Mux : Mux  Inputs=2
  Mux1 : Mux  Inputs=2
  Product : Product  Inputs=3  SaturateOnIntegerOverflow=on  InputSameDT=on  OutDataTypeStr=Inherit: Same as first input
  "Scale Length, ft" : Constant  Value=1750/2
  Ux / U20 : Fcn  Expr=ln(u(1)/.15)/ln(20/.15)
  alt >2000 ft : Switch  Threshold=2000  SaturateOnIntegerOverflow=on  InputSameDT=on
  "ft -> m" : Gain  Gain=.3048  SaturateOnIntegerOverflow=on  OutDataTypeStr=Inherit: Same as input  ParamDataTypeStr=Inherit: Same as input
  "m -> ft" : Gain  Gain=1/.3048  SaturateOnIntegerOverflow=on  OutDataTypeStr=Inherit: Same as input  ParamDataTypeStr=Inherit: Same as input
  "moderate sigma, f/s" : Lookup  InputValues=[2000 12000 44000 100000]  Table=[10 10 3 3]  SaturateOnIntegerOverflow=on
  "severe sigma, f/s" : Lookup  InputValues=[2000 5000 22000 80000 100000]  Table=[15.5 21.5 21.5 3 3]  SaturateOnIntegerOverflow=on
  sigma v/ sigma w1 : Fcn  Expr=(.177+.000823*u(1))^(-.4)
  "sigma, m/s" : Outport
  "scale length, m" : Outport  Port=2
  wires:
  Ux / U20/1 -> Product/2
  MinMax1/1 -> Ux / U20/1
  2/1 -> MinMax1/1
  "0.1*mean wind, fps sigma w = to 2.5f/s * intensity Fig 263, pg 654"/1 -> Product/1
  1/1 -> MinMax/1
  "ft -> m"/1 -> Demux/1
  alt >2000 ft/1 -> "ft -> m"/1
  Demux/1 -> "sigma, m/s"/1
  Demux/2 -> "scale length, m"/1
  L v / sigma w/1 -> Mux1/2
  Mux1/1 -> alt >2000 ft/3
  "m -> ft"/1 -> MinMax1/2, L v / sigma w/1, sigma v/ sigma w1/1, "moderate sigma, f/s"/1, "Light sigma, f/s"/1, "severe sigma, f/s"/1, alt >2000 ft/2
  "Scale Length, ft"/1 -> Mux/2
  intensity/1 -> "0.1*mean wind, fps sigma w = to 2.5f/s * intensity Fig 263, pg 654"/1, Multiport Switch/1
  Mux/1 -> alt >2000 ft/1
  Multiport Switch/1 -> Mux/1
  "alt, m"/1 -> "m -> ft"/1
  "severe sigma, f/s"/1 -> Multiport Switch/4
  "moderate sigma, f/s"/1 -> Multiport Switch/3
  "Light sigma, f/s"/1 -> Multiport Switch/2
  sigma v/ sigma w1/1 -> MinMax/2
  MinMax/1 -> Product/3
  Product/1 -> Mux1/1

== system UserContent_lib/Input Generator/Winds/Turbulence  Model/Dryden Model/Lateral Turbulence/SubSystem1/Tm-4511 severe data ==
  note: "Light" and "Moderate" sigmas are ZERO below 1km alt.
      | Table 2-79 does not define them.
  "alt, m" : Inport
  intensity : Inport  Port=2
  "Lateral sigma, m/s light TM-4511 Table 2-79" : Lookup  InputValues="[10 20 30 40 50 60 70 80 90 100 200 304.8 305 400  762 769 1000 2000 4000 6000 8000 10000 12000 14000 16000]"  Table="[0   0   0   0   0   0   0   0   0    0    0    0   0   0   0   0   .17  .17  .2   .21   .22   .22   .25   .26   .24   ]"  SaturateOnIntegerOverflow=on
  "Lateral sigma, m/s moderate TM-4511 Table 2-79" : Lookup  InputValues="[10 20 30 40 50 60 70 80 90 100 200 304.8 305 400  762 769 1000 2000 4000 6000 8000 10000 12000 14000 16000]"  Table="[0   0  0    0    0   0  0  0   0   0     0    0      0     0      0    0  1.65  1.65 2.04 2.13 2.15 2.23 2.47 2.62 2.44]"  SaturateOnIntegerOverflow=on
  "Lateral sigma, m/s severe TM-4511 Table 2-79" : Lookup  InputValues=[10 20 30 40 50 60 70 80 90 100 200 304.8 305 400 762 769 1000 2000 4000 6000 8000 10000 12000 14000 16000]  Table=[1.67 1.98 2.2 2.36 2.49 2.61 2.71 2.81 2.89 2.97 3.53 3.95 4.37 4.39 4.39 5.7 5.7 5.8 6.24 7.16 7.59 7.72 7.89 6.93 5]  LookUpMeth=Interpolation-Use End Values  SaturateOnIntegerOverflow=on
  "Lateral, Scale, m TM-4511 Table 2-79" : Lookup  InputValues=[0 10 20 30 40 50 60 70 80 90 100 200 304.8 305 762 769 900 1000 2000 4000 6000 8000 10000 12000 14000 16000]  Table=[11 11 19 28 35 42 49 56 63 69 75 134 190 300 300 533 533 832 902 1040 1040 1040 1230 1800 2820 3400]  LookUpMeth=Interpolation-Use End Values  SaturateOnIntegerOverflow=on
  Multiport Switch : MultiPortSwitch  zeroidx=off  SaturateOnIntegerOverflow=on  InputSameDT=on
  "sigma, m/s" : Outport
  "scale length, m" : Outport  Port=2
  wires:
  intensity/1 -> Multiport Switch/1
  "Lateral sigma, m/s light TM-4511 Table 2-79"/1 -> Multiport Switch/2
  "Lateral sigma, m/s moderate TM-4511 Table 2-79"/1 -> Multiport Switch/3
  "Lateral sigma, m/s severe TM-4511 Table 2-79"/1 -> Multiport Switch/4
  Multiport Switch/1 -> "sigma, m/s"/1
  "Lateral, Scale, m TM-4511 Table 2-79"/1 -> "scale length, m"/1
  "alt, m"/1 -> "Lateral sigma, m/s light TM-4511 Table 2-79"/1, "Lateral sigma, m/s moderate TM-4511 Table 2-79"/1, "Lateral, Scale, m TM-4511 Table 2-79"/1, "Lateral sigma, m/s severe TM-4511 Table 2-79"/1

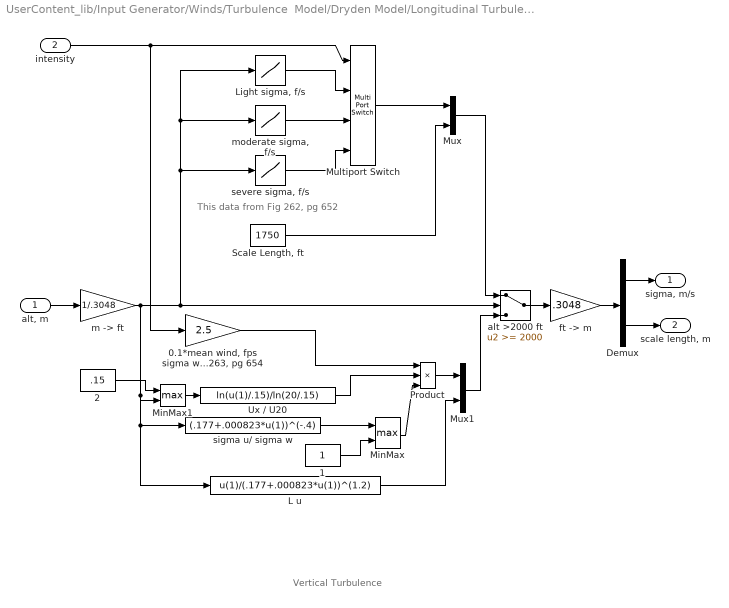
== system UserContent_lib/Input Generator/Winds/Turbulence  Model/Dryden Model/Longitudinal Turbulence/filter parameters/MIL-STD-1797A APPENDIX A  ==
  note: Vertical Turbulence
  note: This data from Fig 262, pg 652
  "alt, m" : Inport
  intensity : Inport  Port=2
  "0.1*mean wind, fps sigma w = to 2.5f/s * intensity Fig 263, pg 654" : Gain  Gain=2.5  SaturateOnIntegerOverflow=on  OutDataTypeStr=Inherit: Same as input  ParamDataTypeStr=Inherit: Same as input
  1 : Constant
  2 : Constant  Value=.15
  Demux : Demux  Outputs=2
  "L u " : Fcn  Expr=u(1)/(.177+.000823*u(1))^(1.2)
  "Light sigma, f/s" : Lookup  InputValues=[2000 9000 18000 100000]  Table=[5 5 3 3]  SaturateOnIntegerOverflow=on
  MinMax : MinMax  Function=max  Inputs=2  SaturateOnIntegerOverflow=on  InputSameDT=on
  MinMax1 : MinMax  Function=max  Inputs=2  SaturateOnIntegerOverflow=on  InputSameDT=on
  Multiport Switch : MultiPortSwitch  zeroidx=off  SaturateOnIntegerOverflow=on  InputSameDT=on
  Mux : Mux  Inputs=2
  Mux1 : Mux  Inputs=2
  Product : Product  Inputs=3  SaturateOnIntegerOverflow=on  InputSameDT=on  OutDataTypeStr=Inherit: Same as first input
  "Scale Length, ft" : Constant  Value=1750
  Ux / U20 : Fcn  Expr=ln(u(1)/.15)/ln(20/.15)
  alt >2000 ft : Switch  Threshold=2000  SaturateOnIntegerOverflow=on  InputSameDT=on
  "ft -> m" : Gain  Gain=.3048  SaturateOnIntegerOverflow=on  OutDataTypeStr=Inherit: Same as input  ParamDataTypeStr=Inherit: Same as input
  "m -> ft" : Gain  Gain=1/.3048  SaturateOnIntegerOverflow=on  OutDataTypeStr=Inherit: Same as input  ParamDataTypeStr=Inherit: Same as input
  "moderate sigma, f/s" : Lookup  InputValues=[2000 12000 44000 100000]  Table=[10 10 3 3]  SaturateOnIntegerOverflow=on
  "severe sigma, f/s" : Lookup  InputValues=[2000 5000 22000 80000 100000]  Table=[15.5 21.5 21.5 3 3]  SaturateOnIntegerOverflow=on
  sigma u/ sigma w : Fcn  Expr=(.177+.000823*u(1))^(-.4)
  "sigma, m/s" : Outport
  "scale length, m" : Outport  Port=2
  wires:
  Ux / U20/1 -> Product/2
  Product/1 -> Mux1/1
  MinMax/1 -> Product/3
  sigma u/ sigma w/1 -> MinMax/1
  1/1 -> MinMax/2
  MinMax1/1 -> Ux / U20/1
  2/1 -> MinMax1/1
  "0.1*mean wind, fps sigma w = to 2.5f/s * intensity Fig 263, pg 654"/1 -> Product/1
  "ft -> m"/1 -> Demux/1
  alt >2000 ft/1 -> "ft -> m"/1
  "L u "/1 -> Mux1/2
  Mux1/1 -> alt >2000 ft/3
  "m -> ft"/1 -> MinMax1/2, "L u "/1, sigma u/ sigma w/1, "moderate sigma, f/s"/1, "Light sigma, f/s"/1, "severe sigma, f/s"/1, alt >2000 ft/2
  Demux/1 -> "sigma, m/s"/1
  Demux/2 -> "scale length, m"/1
  "Scale Length, ft"/1 -> Mux/2
  intensity/1 -> "0.1*mean wind, fps sigma w = to 2.5f/s * intensity Fig 263, pg 654"/1, Multiport Switch/1
  Mux/1 -> alt >2000 ft/1
  Multiport Switch/1 -> Mux/1
  "alt, m"/1 -> "m -> ft"/1
  "severe sigma, f/s"/1 -> Multiport Switch/4
  "moderate sigma, f/s"/1 -> Multiport Switch/3
  "Light sigma, f/s"/1 -> Multiport Switch/2
